simulink model "sampleModel135"  (R2021b)
settings: Solver=VariableStepAuto  StartTime=0.0  StopTime=10.0  RelTol=1e-3
undefined symbols (not defined in the file or in its folder): DiscIntNeverNeededParam, Newton, Raphson
libraries: simulink x19, slpidlib x3
settings Model: Creator=user  LastModifiedBy=user

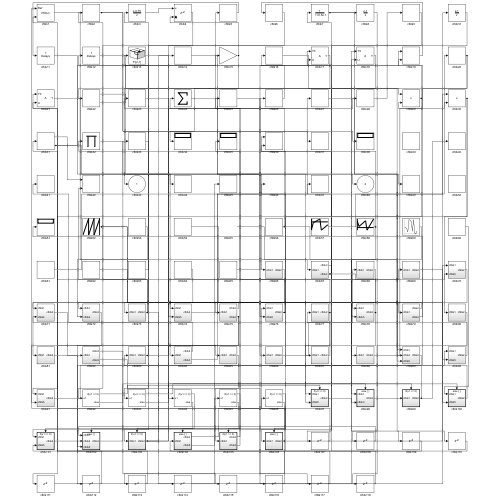
[thumbnail: Simulink's stored preview of the top-level diagram]
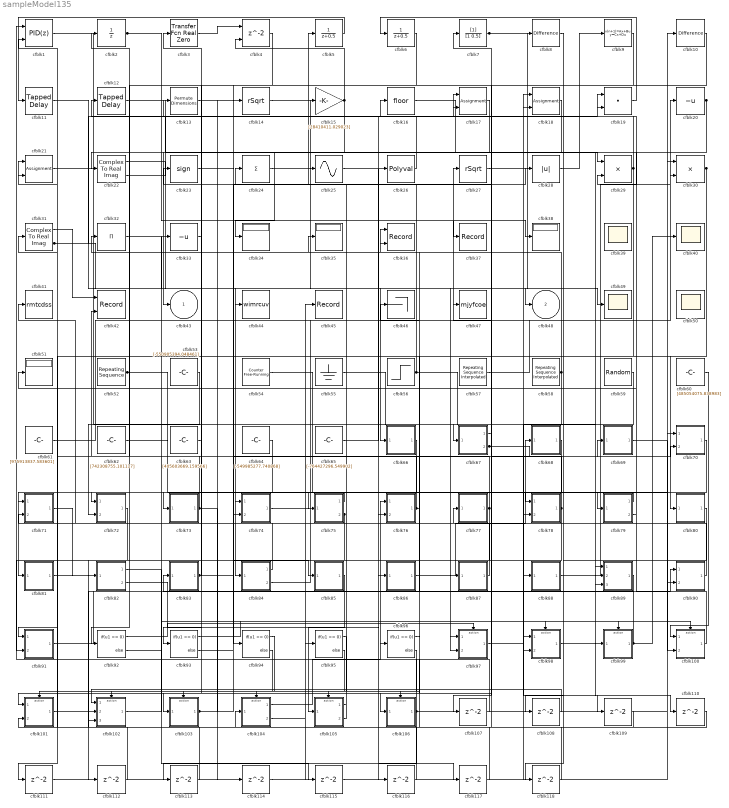
== system sampleModel135 ==
  cfblk1 : slpidlib/PID Controller (2DOF)  Controller=PID  Form=Parallel  TimeDomain=Discrete-time  UseExternalTs=off  SampleTime=1  IntegratorMethod=Forward Euler  FilterMethod=Forward Euler  ControllerParametersSource=internal  P=1  I=1  D=0  UseFilter=on  N=100  b=1  c=1  TunerSelectOption=Transfer Function Based (PID Tuner App)  InitialConditionSource=internal  InitialConditionForIntegrator=0  InitialConditionForFilter=0  DifferentiatorICPrevScaledInput=0  ExternalReset=none  TrackingMode=off  Kt=1  LimitOutput=off  SatLimitsSource=internal  UpperSaturationLimit=inf  LowerSaturationLimit=-inf  LinearizeAsGain=off  AntiWindupMode=none  Kb=1  POutMin=[]  POutMax=[]  IOutMin=[]  IOutMax=[]  DOutMin=[]  DOutMax=[]  NOutMin=[]  NOutMax=[]  bOutMin=[]  bOutMax=[]  cOutMin=[]  cOutMax=[]  SumOutMin=[]  SumOutMax=[]  SaturationOutMin=[]  SaturationOutMax=[]  PParamMin=[]  PParamMax=[]  IParamMin=[]  IParamMax=[]  DParamMin=[]  DParamMax=[]  NParamMin=[]  NParamMax=[]  bParamMin=[]  bParamMax=[]  cParamMin=[]  cParamMax=[]  KbParamMin=[]  KbParamMax=[]  KtParamMin=[]  KtParamMax=[]  KbOutMin=[]  KbOutMax=[]  KtOutMin=[]  KtOutMax=[]  IntegratorOutMin=[]  IntegratorOutMax=[]  FilterOutMin=[]  FilterOutMax=[]  SumI1OutMin=[]  SumI1OutMax=[]  SumI2OutMin=[]  SumI2OutMax=[]  SumI3OutMin=[]  SumI3OutMax=[]  SumI4OutMin=[]  SumI4OutMax=[]  SumDOutMin=[]  SumDOutMax=[]  Sum1OutMin=[]  Sum1OutMax=[]  Sum2OutMin=[]  Sum2OutMax=[]  Sum3OutMin=[]  Sum3OutMax=[]  DifferentiatorOutMin=[]  DifferentiatorOutMax=[]  FilterDiffOutCoefMin=[]  FilterDiffOutCoefMax=[]  ReciprocalOutMin=[]  ReciprocalOutMax=[]  SumDenOutMin=[]  SumDenOutMax=[]  SumNumOutMin=[]  SumNumOutMax=[]  DivideOutMin=[]  DivideOutMax=[]  UdiffTsProdOutMin=[]  UdiffTsProdOutMax=[]  NTsProdOutMin=[]  NTsProdOutMax=[]  UintegralTsProdOutMin=[]  UintegralTsProdOutMax=[]  UngainTsProdOutMin=[]  UngainTsProdOutMax=[]  IntegratorContinuousStateAttributes=''  IntegratorStateMustResolveToSignalObject=off  IntegratorRTWStateStorageClass=Auto  FilterContinuousStateAttributes=''  FilterStateMustResolveToSignalObject=off  FilterRTWStateStorageClass=Auto  ParallelPVariant=InternalParameters  IdealPVariant=Disabled  IVariant=InternalParameters  DVariant=InternalParameters  bVariant=InternalParameters  cVariant=InternalParameters  IntegratorVariant=Discrete  SatVariant=Disabled  AWVariant=Passthrough  PCopyVariant=Disabled  TRVariant=Disabled  FdbkBlocksVariant=Forward  IdealPFdbkVariant=Disabled  SatFdbkVariant=Disabled  DerivativeFilterVariant=ForwardEulerFilter  NVariant=InternalParameters  NCopyVariant=Disabled  FilterICVariant=InternalICsFilter  IntegratorICVariant=InternalICs  ExternalResetVariant=Disabled  TRSumVariant=Passthrough  SumFdbkVariant=Disabled  SumVariant=Sum_PID  TsampFilterVariant=InternalTs  TsampNgainVariant=Passthrough  TsampIntegralVariant=Passthrough  ExternalSaturationOutDataTypeStr=Inherit: Same as second input
      settings: SourceProductBaseCode=SL
  cfblk10 : simulink/Discrete/Difference  ICPrevInput=0.0  OutMin=[]  OutMax=[]  OutDataTypeStr=Inherit: Inherit via back propagation  OutDataType=fixdt(1, 16)  OutScaling=2^-10  DoSatur=off
  cfblk100 : Subsystem  TreatAsAtomicUnit=on
  cfblk101 : Subsystem  TreatAsAtomicUnit=on
  cfblk102 : Subsystem  TreatAsAtomicUnit=on
  cfblk103 : Subsystem  TreatAsAtomicUnit=on
  cfblk104 : Subsystem  TreatAsAtomicUnit=on
  cfblk105 : Subsystem  TreatAsAtomicUnit=on
  cfblk106 : Subsystem  TreatAsAtomicUnit=on
  cfblk{107..118} (12 alike) : Delay  SampleTime=1
  cfblk11 : simulink/Discrete/Tapped Delay  vinit=0.0  samptime=-1  NumDelays=1  DelayOrder=Oldest  includeCurrent=off
  cfblk12 : simulink/Discrete/Tapped Delay  vinit=0.0  samptime=-1  NumDelays=1  DelayOrder=Oldest  includeCurrent=off
  cfblk13 : PermuteDimensions
  cfblk14 : Sqrt  Operator=rSqrt  AlgorithmType=Newton-Raphson  SaturateOnIntegerOverflow=on
  cfblk15 : Gain  Gain=[28410411.029023]
  cfblk16 : Rounding
  cfblk17 : Assignment  DiagnosticForDimensions=Warning  IndexOptions=Index vector (dialog)  Indices=1  OutputSizes=1
  cfblk18 : Assignment  DiagnosticForDimensions=Warning  IndexOptions=Index vector (dialog)  Indices=1  OutputSizes=1
  cfblk19 : DotProduct  InputSameDT=on  OutDataTypeStr=Inherit: Inherit via internal rule
  cfblk2 : UnitDelay  HasFrameUpgradeWarning=on
  cfblk20 : UnaryMinus
  cfblk21 : Assignment  DiagnosticForDimensions=Warning  IndexOptions=Index vector (dialog)  Indices=1  OutputSizes=1
  cfblk22 : ComplexToRealImag
  cfblk23 : Signum
  cfblk24 : Sum  Inputs=+
  cfblk25 : Sin  TimeSource=Use external signal  SampleTime=0
  cfblk26 : Polyval  Coefs=[ +2.081618890e-019, -1.441693666e-014, +4.719686976e-010, -8.536869453e-006, +1.621573104e-001, -8.087801117e+001 ]
  cfblk27 : Sqrt  Operator=rSqrt  AlgorithmType=Newton-Raphson  SaturateOnIntegerOverflow=on
  cfblk28 : Abs
  cfblk29 : Product  Inputs=**
  cfblk3 : simulink/Discrete/Transfer Fcn Real Zero  ZeroZ=0.75  ICPrevInput=0.0  DoSatur=off
      settings: SourceProductBaseCode=SL
  cfblk30 : Product
  cfblk31 : ComplexToRealImag
  cfblk32 : Product  Inputs=*
  cfblk33 : UnaryMinus
  cfblk{34..35,38,51} (4 alike) : Display
  cfblk36 : Record  FileSettingsInternal="{\"entries\":[{\"content\":{\"excelSettings\":{\"content\":{},\"type\":\"Streamout.ExcelSettings\"}},\"type\":\"Streamout.FileSettingStorage\",\"uuid\":\"dc4603f7-060f-47ee-a389-6b2f5d8eacf3\"}],\"packageUris\":[\"http://schema.mathworks.com/mf0/streamout_blocks/R2020a\"],\"version\":\"1.0\"}"  Layout=[1 1]  SignalsInternal="{\"entries\":[{\"content\":{\"signals\":[{\"content\":{\"blockPath\":[\"sampleModel135/cfblk36\"],\"channel\":[],\"dimensions\":[1],\"domain\":\"sampleModel135/cfblk36\",\"lineColor\":\"#a2142f\",\"plots\":[1],\"port\":1,\"sid\":[\"\"],\"signalID\":4712,\"signalName\":\"cfblk76\"},\"type\":\"RecordBlkView.Signal\",\"uuid\":\"88f8ffe8-7962-43a1-8896-d692d2f87f4c\"},{\"content\":{\"blockPath\":[\"sampleModel135/cfblk36\"],\"channel\":[],\"dimensions\":[1],\"domain\":\"sampleModel135/cfblk36\",\"lineColor\":\"#139fff\",\"plots\":[1],\"port\":2,\"sid\":[\"\"],\"signalID\":4716,\"signalName\":\"cfblk67:2\"},\"type\":\"RecordBlkView.Signal\",\"uuid\":\"a67d97e2-9e96-4cb3-bdb1-be52fcd4c5cb\"}]},\"type\":\"RecordBlkView.InputSignals\",\"uuid\":\"0687f38a-ff4e-4925-8716-18ef31107799\"}],\"packageUris\":[\"http://schema.mathworks.com/mf0/streamout_blocks/R2020a\"],\"version\":\"1.0\"}"  VisualizationBindings="{\"xyplotplugin\":{\"info\":[{\"series\":[{\"bindingParametersList\":[{\"parameter\":\"X-Axis\",\"signalID\":4712,\"signalName\":\"cfblk76\"},{\"parameter\":\"Y-Axis\",\"signalID\":4716,\"signalName\":\"cfblk67:2\"}],\"seriesID\":6412}],\"subplotID\":1}]}}"  CompatibilityTag=XY
  cfblk37 : Record  FileSettingsInternal="{\"entries\":[{\"content\":{\"excelSettings\":{\"content\":{},\"type\":\"Streamout.ExcelSettings\"}},\"type\":\"Streamout.FileSettingStorage\",\"uuid\":\"5de6cc85-0c80-4659-8aff-d8a8f7568a02\"}],\"packageUris\":[\"http://schema.mathworks.com/mf0/streamout_blocks/R2020a\"],\"version\":\"1.0\"}"  SignalsInternal="{\"entries\":[{\"content\":{\"signals\":[{\"content\":{\"blockPath\":[\"sampleModel135/cfblk37\"],\"channel\":[],\"dimensions\":[1],\"domain\":\"sampleModel135/cfblk37\",\"lineColor\":\"#a2142f\",\"plots\":[1],\"port\":1,\"sid\":[\"\"],\"signalID\":4720,\"signalName\":\"cfblk2\"},\"type\":\"RecordBlkView.Signal\",\"uuid\":\"9ad653bb-3f93-4fe3-8d88-ee341a26a170\"}]},\"type\":\"RecordBlkView.InputSignals\",\"uuid\":\"e2ea3720-dc8c-4658-944f-b29d6f1fb988\"}],\"packageUris\":[\"http://schema.mathworks.com/mf0/streamout_blocks/R2020a\"],\"version\":\"1.0\"}"  VisualizationBindings="{\"sparklinesplugin\":{\"info\":[{\"bindingParametersList\":[],\"subplotID\":1}]}}"
  cfblk{39..40,49..50} (4 alike) : Scope
      cfblk39 settings: Floating=on
      cfblk50 settings: Floating=on
  cfblk4 : Delay  ShowEnablePort=on  SampleTime=1
      settings: InputPortMap=u0,e6
  cfblk41 : ToWorkspace  VariableName=rmtcdss  SaveFormat=Timeseries  SampleTime=-1
  cfblk42 : Record  FileSettingsInternal="{\"entries\":[{\"content\":{\"excelSettings\":{\"content\":{},\"type\":\"Streamout.ExcelSettings\"}},\"type\":\"Streamout.FileSettingStorage\",\"uuid\":\"3a613f90-b4b9-4c61-961a-fdb05aa120f1\"}],\"packageUris\":[\"http://schema.mathworks.com/mf0/streamout_blocks/R2020a\"],\"version\":\"1.0\"}"  Layout=[1 1]  SignalsInternal="{\"entries\":[{\"content\":{\"signals\":[{\"content\":{\"blockPath\":[\"sampleModel135/cfblk42\"],\"channel\":[],\"dimensions\":[1],\"domain\":\"sampleModel135/cfblk42\",\"lineColor\":\"#a2142f\",\"plots\":[1],\"port\":1,\"sid\":[\"\"],\"signalID\":4724,\"signalName\":\"cfblk31:1\"},\"type\":\"RecordBlkView.Signal\",\"uuid\":\"ce349fb7-b3a0-4447-98f3-427877e07b8c\"},{\"content\":{\"blockPath\":[\"sampleModel135/cfblk42\"],\"channel\":[],\"dimensions\":[1],\"domain\":\"sampleModel135/cfblk42\",\"lineColor\":\"#139fff\",\"plots\":[1],\"port\":2,\"sid\":[\"\"],\"signalID\":4728,\"signalName\":\"cfblk73\"},\"type\":\"RecordBlkView.Signal\",\"uuid\":\"6a64b2c5-78f2-443e-96fe-3bc98703bc06\"}]},\"type\":\"RecordBlkView.InputSignals\",\"uuid\":\"472f762d-471a-4371-944a-d30467dc95ae\"}],\"packageUris\":[\"http://schema.mathworks.com/mf0/streamout_blocks/R2020a\"],\"version\":\"1.0\"}"  VisualizationBindings="{\"xyplotplugin\":{\"info\":[{\"series\":[{\"bindingParametersList\":[{\"parameter\":\"X-Axis\",\"signalID\":4724,\"signalName\":\"cfblk31:1\"},{\"parameter\":\"Y-Axis\",\"signalID\":4728,\"signalName\":\"cfblk73\"}],\"seriesID\":39813}],\"subplotID\":1}]}}"  CompatibilityTag=XY
  cfblk44 : ToWorkspace  VariableName=wimrcuv  SaveFormat=Timeseries  SampleTime=-1
  cfblk45 : Record  FileSettingsInternal="{\"entries\":[{\"content\":{\"excelSettings\":{\"content\":{},\"type\":\"Streamout.ExcelSettings\"}},\"type\":\"Streamout.FileSettingStorage\",\"uuid\":\"b06d5a54-4607-4223-bf0d-fc84dbd604d8\"}],\"packageUris\":[\"http://schema.mathworks.com/mf0/streamout_blocks/R2020a\"],\"version\":\"1.0\"}"  SignalsInternal="{\"entries\":[{\"content\":{\"signals\":[{\"content\":{\"blockPath\":[\"sampleModel135/cfblk45\"],\"channel\":[],\"dimensions\":[1],\"domain\":\"sampleModel135/cfblk45\",\"lineColor\":\"#b746ff\",\"plots\":[1],\"port\":1,\"sid\":[\"\"],\"signalID\":4732,\"signalName\":\"cfblk104:2\"},\"type\":\"RecordBlkView.Signal\",\"uuid\":\"831cb24a-ecf3-4b9e-81f9-60f1a74fc749\"}]},\"type\":\"RecordBlkView.InputSignals\",\"uuid\":\"5b04a1d9-3887-4891-afc8-c46e7e218a24\"}],\"packageUris\":[\"http://schema.mathworks.com/mf0/streamout_blocks/R2020a\"],\"version\":\"1.0\"}"  VisualizationBindings="{\"sparklinesplugin\":{\"info\":[{\"bindingParametersList\":[],\"subplotID\":1}]}}"
  cfblk46 : Terminator
  cfblk47 : ToWorkspace  VariableName=mjyfcoe  SaveFormat=Timeseries  SampleTime=-1
  cfblk5 : DiscreteTransferFcn  SampleTime=1
  cfblk52 : simulink/Sources/Repeating Sequence  rep_seq_t=[0 2]  rep_seq_y=[477640940.241571, 909947082.671190]
  cfblk53 : Constant  Value=[-550905394.048461]  SampleTime=1
  cfblk54 : simulink/Sources/Counter Free-Running  NumBits=[15.000000]  tsamp=-1
  cfblk55 : Ground
  cfblk56 : Step  Time=[24.000000]  Before=[-595461991.186605]  After=[-347251148.629385]  SampleTime=0
  cfblk57 : simulink/Sources/Repeating Sequence Interpolated  OutValues=[-698628012.134013, -76558517.748631, 311619998.084971, -846087687.549569, -298956944.646346]  TimeValues=[0 0.1 0.5 0.6 1].'  LookUpMeth=Interpolation-Use End Values  tsamp=0.01  OutMin=[]  OutMax=[]  OutDataTypeStr=double  OutputDataTypeScalingMode=double  OutDataType=fixdt(0,8)  OutScaling=2^-10
  cfblk58 : simulink/Sources/Repeating Sequence Interpolated  OutValues=[752332312.195068, 107819467.006181, 768088279.352811, -288841479.675765, 972343704.108739]  TimeValues=[0 0.1 0.5 0.6 1].'  LookUpMeth=Use Input Above  tsamp=0.01  OutMin=[]  OutMax=[]  OutDataTypeStr=double  OutputDataTypeScalingMode=double  OutDataType=fixdt(0,8)  OutScaling=2^-10
  cfblk59 : RandomNumber  Mean=[72182.026536]  Variance=[16955.399432]  Seed=[307408944.000000]  SampleTime=0.1
  cfblk6 : DiscreteTransferFcn  SampleTime=1
  cfblk60 : Constant  Value=[485054075.838983]  SampleTime=1
  cfblk61 : Constant  Value=[975913837.583601]  SampleTime=1
  cfblk62 : Constant  Value=[742308755.101117]  SampleTime=1
  cfblk63 : Constant  Value=[405603669.159566]  SampleTime=1
  cfblk64 : Constant  Value=[-549985277.740868]  SampleTime=1
  cfblk65 : Constant  Value=[-764427296.549902]  SampleTime=1
  cfblk66 : Subsystem
  cfblk67 : Subsystem
  cfblk68 : Subsystem
  cfblk69 : Subsystem
  cfblk7 : DiscreteFilter  SampleTime=1
  cfblk70 : Subsystem
  cfblk71 : Subsystem
  cfblk72 : Subsystem
  cfblk73 : Subsystem
  cfblk74 : Subsystem
  cfblk75 : Subsystem
  cfblk76 : Subsystem
  cfblk77 : Subsystem
  cfblk78 : Subsystem
  cfblk79 : Subsystem
  cfblk8 : simulink/Discrete/Difference  ICPrevInput=0.0  OutMin=[]  OutMax=[]  OutDataTypeStr=Inherit: Inherit via back propagation  OutDataType=fixdt(1, 16)  OutScaling=2^-10  DoSatur=off
  cfblk80 : Subsystem
  cfblk81 : Subsystem
  cfblk82 : Subsystem
  cfblk83 : Subsystem
  cfblk84 : Subsystem
  cfblk85 : Subsystem
  cfblk86 : Subsystem
  cfblk87 : Subsystem
  cfblk88 : Subsystem
  cfblk89 : Subsystem
  cfblk9 : DiscreteStateSpace
  cfblk90 : Subsystem
  cfblk91 : Subsystem
  cfblk{92..96} (5 alike) : If  IfExpression=u1 >= 0  SampleTime=1
  cfblk97 : Subsystem  TreatAsAtomicUnit=on
  cfblk98 : Subsystem  TreatAsAtomicUnit=on
  cfblk99 : Subsystem  TreatAsAtomicUnit=on
  cfblk43 : Outport
  cfblk48 : Outport  Port=2
  wires:
  cfblk71/1(cfblk2) -> cfblk82/1(cfblk1)
  cfblk17/1 -> cfblk43/1
  cfblk28/1 -> cfblk9/1
  cfblk18/1 -> cfblk24/1
  cfblk84/1(cfblk2) -> cfblk41/1
  cfblk15/1 -> cfblk34/1, cfblk4/2
  cfblk89/1(cfblk2) -> cfblk83/1(cfblk1)
  cfblk85/1(cfblk2) -> cfblk105/1(cfblk1)
  cfblk1/1 -> cfblk67/1(cfblk1)
  cfblk5/1 -> cfblk11/1
  cfblk19/1 -> cfblk6/1
  cfblk90/1(cfblk2) -> cfblk77/1(cfblk1)
  cfblk68/1(cfblk2) -> cfblk81/1(cfblk1)
  cfblk61/1 -> cfblk27/1
  cfblk12/1 -> cfblk29/1
  cfblk56/1 -> cfblk5/1, cfblk89/3(cfblk5)
  cfblk101/1(cfblk2) -> cfblk90/1(cfblk1)
  cfblk13/1 -> cfblk94/1
  cfblk22/1 -> cfblk84/1(cfblk1)
  cfblk83/1(cfblk2) -> cfblk3/1, cfblk85/1(cfblk1)
  cfblk64/1 -> cfblk72/1(cfblk1)
  cfblk62/1 -> cfblk97/1(cfblk1)
  cfblk104/1(cfblk2) -> cfblk76/1(cfblk1)
  cfblk30/1 -> cfblk80/1(cfblk1), cfblk111/1
  cfblk20/1 -> cfblk29/2, cfblk22/1
  cfblk86/1(cfblk2) -> cfblk68/1(cfblk1)
  cfblk53/1 -> cfblk72/2(cfblk4)
  cfblk102/1(cfblk2) -> cfblk33/1
  cfblk29/1 -> cfblk16/1, cfblk106/1(cfblk1)
  cfblk88/1(cfblk2) -> cfblk20/1
  cfblk104/2(cfblk5) -> cfblk45/1
  cfblk16/1 -> cfblk99/1(cfblk1)
  cfblk31/1 -> cfblk42/1
  cfblk21/1 -> cfblk87/1(cfblk1)
  cfblk23/1 -> cfblk79/1(cfblk1)
  cfblk66/1(cfblk2) -> cfblk71/1(cfblk1)
  cfblk73/1(cfblk2) -> cfblk12/1, cfblk42/2, cfblk114/1
  cfblk60/1 -> cfblk100/1(cfblk1)
  cfblk11/1 -> cfblk44/1
  cfblk52/1 -> cfblk76/2(cfblk5), cfblk98/1(cfblk1)
  cfblk24/1 -> cfblk66/1(cfblk1)
  cfblk14/1 -> cfblk48/1
  cfblk106/1(cfblk2) -> cfblk30/1, cfblk21/1, cfblk113/1
  cfblk76/1(cfblk2) -> cfblk36/1, cfblk35/1
  cfblk63/1 -> cfblk13/1
  cfblk27/1 -> cfblk89/1(cfblk1)
  cfblk100/1(cfblk2) -> cfblk19/1
  cfblk33/1 -> cfblk93/1
  cfblk78/1(cfblk2) -> cfblk97/2(cfblk5), cfblk47/1
  cfblk22/2 -> cfblk15/1
  cfblk105/1(cfblk2) -> cfblk25/1
  cfblk67/1(cfblk2) -> cfblk101/1(cfblk1)
  cfblk74/1(cfblk2) -> cfblk10/1
  cfblk99/1(cfblk2) -> cfblk46/1, cfblk40/1
  cfblk7/1 -> cfblk89/2(cfblk4), cfblk8/1
  cfblk79/1(cfblk2) -> cfblk78/1(cfblk1)
  cfblk67/2(cfblk4) -> cfblk36/2, cfblk69/1(cfblk1), cfblk17/2
  cfblk57/1 -> cfblk30/2
  cfblk72/1(cfblk2) -> cfblk102/3(cfblk5)
  cfblk69/1(cfblk2) -> cfblk90/2(cfblk5)
  cfblk84/2(cfblk3) -> cfblk26/1
  cfblk91/1(cfblk2) -> cfblk18/1
  cfblk105/2(cfblk4) -> cfblk23/1
  cfblk10/1 -> cfblk73/1(cfblk1)
  cfblk79/2(cfblk4) -> cfblk51/1
  cfblk75/1(cfblk2) -> cfblk74/1(cfblk1)
  cfblk26/1 -> cfblk2/1
  cfblk3/1 -> cfblk4/1
  cfblk2/1 -> cfblk37/1, cfblk38/1
  cfblk87/1(cfblk2) -> cfblk31/1
  cfblk4/1 -> cfblk74/2(cfblk5)
  cfblk31/2 -> cfblk86/1(cfblk1), cfblk19/2
  cfblk70/1(cfblk2) -> cfblk75/1(cfblk1)
  cfblk75/2(cfblk4) -> cfblk91/1(cfblk1), cfblk91/2(cfblk5)
  cfblk77/1(cfblk2) -> cfblk103/1(cfblk1), cfblk21/2
  cfblk55/1 -> cfblk88/1(cfblk1)
  cfblk58/1 -> cfblk32/1, cfblk98/2(cfblk3)
  cfblk54/1 -> cfblk100/2(cfblk5)
  cfblk6/1 -> cfblk92/1
  cfblk59/1 -> cfblk78/2(cfblk5)
  cfblk103/1(cfblk2) -> cfblk28/1, cfblk14/1, cfblk70/2(cfblk5)
  cfblk32/1 -> cfblk49/1
  cfblk65/1 -> cfblk17/1
  cfblk92/1 -> cfblk97/Action
  cfblk92/2 -> cfblk98/Action
  cfblk93/1 -> cfblk99/Action
  cfblk93/2 -> cfblk100/Action
  cfblk94/1 -> cfblk101/Action
  cfblk94/2 -> cfblk102/Action
  cfblk95/1 -> cfblk103/Action
  cfblk95/2 -> cfblk104/Action
  cfblk96/1 -> cfblk105/Action
  cfblk96/2 -> cfblk106/Action
  cfblk9/1 -> cfblk107/1
  cfblk107/1 -> cfblk1/1
  cfblk80/1(cfblk2) -> cfblk108/1
  cfblk108/1 -> cfblk102/1(cfblk1)
  cfblk97/1(cfblk2) -> cfblk109/1
  cfblk109/1 -> cfblk101/2(cfblk5)
  cfblk98/1(cfblk2) -> cfblk110/1
  cfblk110/1 -> cfblk104/1(cfblk1)
  cfblk111/1 -> cfblk95/1
  cfblk81/1(cfblk2) -> cfblk112/1
  cfblk112/1 -> cfblk102/2(cfblk4)
  cfblk113/1 -> cfblk1/2
  cfblk114/1 -> cfblk70/1(cfblk1)
  cfblk82/1(cfblk2) -> cfblk115/1
  cfblk115/1 -> cfblk18/2
  cfblk82/2(cfblk5) -> cfblk116/1
  cfblk116/1 -> cfblk71/2(cfblk4)
  cfblk25/1 -> cfblk117/1
  cfblk117/1 -> cfblk96/1
  cfblk8/1 -> cfblk118/1
  cfblk118/1 -> cfblk7/1

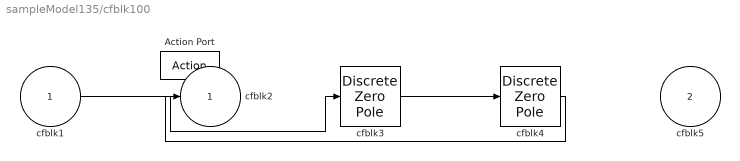
== system sampleModel135/cfblk100 ==
  cfblk1 : Inport
  cfblk5 : Inport  Port=2
  Action Port : ActionPort  ActionPortLabel=else
  cfblk3 : DiscreteZeroPole  Poles=[0 0.5]  Gain=1  SampleTime=-1
  cfblk4 : DiscreteZeroPole  Poles=[0 0.5]  Gain=1  SampleTime=-1
  cfblk2 : Outport
  wires:
  cfblk3/1 -> cfblk4/1
  cfblk1/1 -> cfblk3/1
  cfblk4/1 -> cfblk2/1

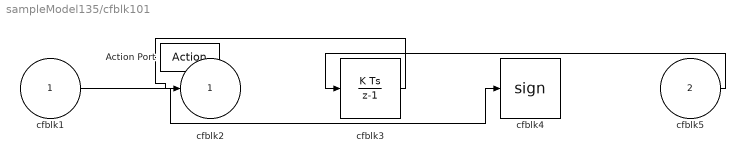
== system sampleModel135/cfblk101 ==
  cfblk1 : Inport
  cfblk5 : Inport  Port=2
  Action Port : ActionPort  ActionPortLabel=if(u1 >= 0)
  cfblk3 : DiscreteIntegrator  SampleTime=-1  ICPrevOutput=DiscIntNeverNeededParam  ICPrevScaledInput=DiscIntNeverNeededParam
  cfblk4 : Signum
  cfblk2 : Outport
  wires:
  cfblk1/1 -> cfblk4/1
  cfblk3/1 -> cfblk2/1
  cfblk5/1 -> cfblk3/1

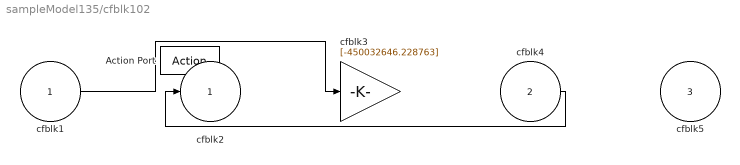
== system sampleModel135/cfblk102 ==
  cfblk1 : Inport
  cfblk4 : Inport  Port=2
  cfblk5 : Inport  Port=3
  Action Port : ActionPort  ActionPortLabel=else
  cfblk3 : Gain  Gain=[-450032646.228763]
  cfblk2 : Outport
  wires:
  cfblk4/1 -> cfblk2/1
  cfblk1/1 -> cfblk3/1

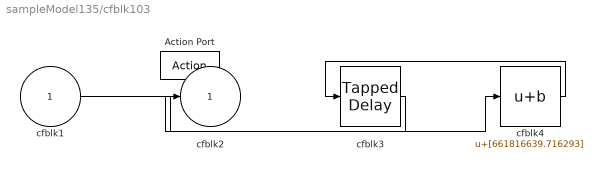
== system sampleModel135/cfblk103 ==
  cfblk1 : Inport
  Action Port : ActionPort  ActionPortLabel=if(u1 >= 0)
  cfblk3 : simulink/Discrete/Tapped Delay  vinit=0.0  samptime=-1  NumDelays=1  DelayOrder=Oldest  includeCurrent=off
  cfblk4 : Bias  Bias=[661816639.716293]
  cfblk2 : Outport
  wires:
  cfblk1/1 -> cfblk4/1
  cfblk4/1 -> cfblk3/1
  cfblk3/1 -> cfblk2/1

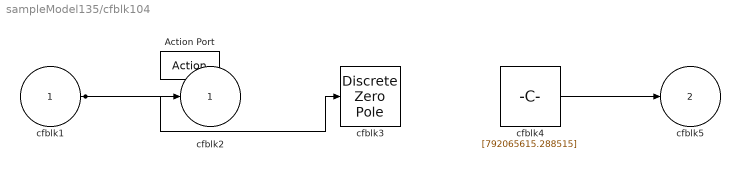
== system sampleModel135/cfblk104 ==
  cfblk1 : Inport
  Action Port : ActionPort  ActionPortLabel=else
  cfblk3 : DiscreteZeroPole  Poles=[0 0.5]  Gain=1  SampleTime=-1
  cfblk4 : Constant  Value=[792065615.288515]  SampleTime=1
  cfblk2 : Outport
  cfblk5 : Outport  Port=2
  wires:
  cfblk4/1 -> cfblk5/1
  cfblk1/1 -> cfblk2/1, cfblk3/1

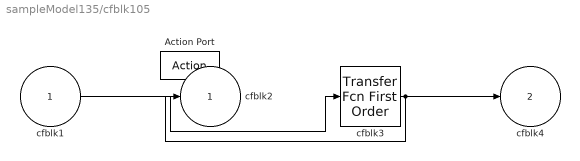
== system sampleModel135/cfblk105 ==
  cfblk1 : Inport
  Action Port : ActionPort  ActionPortLabel=if(u1 >= 0)
  cfblk3 : simulink/Discrete/Transfer Fcn First Order  PoleZ=0.95  ICPrevOutput=0.0  DoSatur=off
  cfblk2 : Outport
  cfblk4 : Outport  Port=2
  wires:
  cfblk1/1 -> cfblk3/1
  cfblk3/1 -> cfblk2/1, cfblk4/1

== system sampleModel135/cfblk106 ==
  cfblk1 : Inport
  Action Port : ActionPort  ActionPortLabel=else
  cfblk3 : ComplexToMagnitudeAngle
  cfblk2 : Outport
  wires:
  cfblk1/1 -> cfblk2/1, cfblk3/1

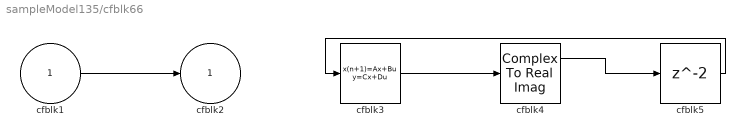
== system sampleModel135/cfblk66 ==
  cfblk1 : Inport
  cfblk3 : DiscreteStateSpace
  cfblk4 : ComplexToRealImag
  cfblk5 : Delay  SampleTime=1
  cfblk2 : Outport
  wires:
  cfblk3/1 -> cfblk4/1
  cfblk1/1 -> cfblk2/1
  cfblk4/1 -> cfblk5/1
  cfblk5/1 -> cfblk3/1

== system sampleModel135/cfblk67 ==
  cfblk1 : Inport
  cfblk3 : DiscreteStateSpace
  cfblk2 : Outport
  cfblk4 : Outport  Port=2
  wires:
  cfblk1/1 -> cfblk4/1, cfblk3/1
  cfblk3/1 -> cfblk2/1

== system sampleModel135/cfblk68 ==
  cfblk1 : Inport
  cfblk3 : DiscreteFilter  SampleTime=1
  cfblk4 : DiscreteFilter  SampleTime=1
  cfblk2 : Outport
  wires:
  cfblk4/1 -> cfblk3/1
  cfblk1/1 -> cfblk4/1
  cfblk3/1 -> cfblk2/1

== system sampleModel135/cfblk69 ==
  cfblk1 : Inport
  cfblk3 : Delay  DelayLengthSource=Input port  SampleTime=1
      settings: InputPortMap=u0,p1
  cfblk2 : Outport
  wires:
  cfblk1/1 -> cfblk3/1, cfblk3/2
  cfblk3/1 -> cfblk2/1

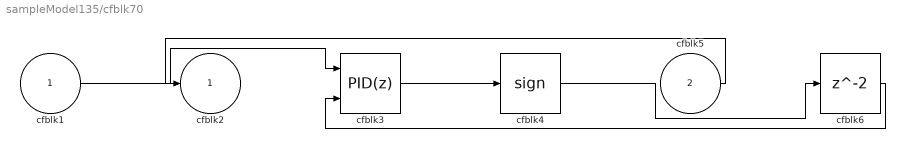
== system sampleModel135/cfblk70 ==
  cfblk1 : Inport
  cfblk5 : Inport  Port=2
  cfblk3 : slpidlib/PID Controller (2DOF)  Controller=PID  Form=Parallel  TimeDomain=Discrete-time  UseExternalTs=off  SampleTime=1  IntegratorMethod=Forward Euler  FilterMethod=Forward Euler  ControllerParametersSource=internal  P=1  I=1  D=0  UseFilter=on  N=100  b=1  c=1  TunerSelectOption=Transfer Function Based (PID Tuner App)  InitialConditionSource=internal  InitialConditionForIntegrator=0  InitialConditionForFilter=0  DifferentiatorICPrevScaledInput=0  ExternalReset=none  TrackingMode=off  Kt=1  LimitOutput=off  SatLimitsSource=internal  UpperSaturationLimit=inf  LowerSaturationLimit=-inf  LinearizeAsGain=off  AntiWindupMode=none  Kb=1  POutMin=[]  POutMax=[]  IOutMin=[]  IOutMax=[]  DOutMin=[]  DOutMax=[]  NOutMin=[]  NOutMax=[]  bOutMin=[]  bOutMax=[]  cOutMin=[]  cOutMax=[]  SumOutMin=[]  SumOutMax=[]  SaturationOutMin=[]  SaturationOutMax=[]  PParamMin=[]  PParamMax=[]  IParamMin=[]  IParamMax=[]  DParamMin=[]  DParamMax=[]  NParamMin=[]  NParamMax=[]  bParamMin=[]  bParamMax=[]  cParamMin=[]  cParamMax=[]  KbParamMin=[]  KbParamMax=[]  KtParamMin=[]  KtParamMax=[]  KbOutMin=[]  KbOutMax=[]  KtOutMin=[]  KtOutMax=[]  IntegratorOutMin=[]  IntegratorOutMax=[]  FilterOutMin=[]  FilterOutMax=[]  SumI1OutMin=[]  SumI1OutMax=[]  SumI2OutMin=[]  SumI2OutMax=[]  SumI3OutMin=[]  SumI3OutMax=[]  SumI4OutMin=[]  SumI4OutMax=[]  SumDOutMin=[]  SumDOutMax=[]  Sum1OutMin=[]  Sum1OutMax=[]  Sum2OutMin=[]  Sum2OutMax=[]  Sum3OutMin=[]  Sum3OutMax=[]  DifferentiatorOutMin=[]  DifferentiatorOutMax=[]  FilterDiffOutCoefMin=[]  FilterDiffOutCoefMax=[]  ReciprocalOutMin=[]  ReciprocalOutMax=[]  SumDenOutMin=[]  SumDenOutMax=[]  SumNumOutMin=[]  SumNumOutMax=[]  DivideOutMin=[]  DivideOutMax=[]  UdiffTsProdOutMin=[]  UdiffTsProdOutMax=[]  NTsProdOutMin=[]  NTsProdOutMax=[]  UintegralTsProdOutMin=[]  UintegralTsProdOutMax=[]  UngainTsProdOutMin=[]  UngainTsProdOutMax=[]  IntegratorContinuousStateAttributes=''  IntegratorStateMustResolveToSignalObject=off  IntegratorRTWStateStorageClass=Auto  FilterContinuousStateAttributes=''  FilterStateMustResolveToSignalObject=off  FilterRTWStateStorageClass=Auto  ParallelPVariant=InternalParameters  IdealPVariant=Disabled  IVariant=InternalParameters  DVariant=InternalParameters  bVariant=InternalParameters  cVariant=InternalParameters  IntegratorVariant=Discrete  SatVariant=Disabled  AWVariant=Passthrough  PCopyVariant=Disabled  TRVariant=Disabled  FdbkBlocksVariant=Forward  IdealPFdbkVariant=Disabled  SatFdbkVariant=Disabled  DerivativeFilterVariant=ForwardEulerFilter  NVariant=InternalParameters  NCopyVariant=Disabled  FilterICVariant=InternalICsFilter  IntegratorICVariant=InternalICs  ExternalResetVariant=Disabled  TRSumVariant=Passthrough  SumFdbkVariant=Disabled  SumVariant=Sum_PID  TsampFilterVariant=InternalTs  TsampNgainVariant=Passthrough  TsampIntegralVariant=Passthrough  ExternalSaturationOutDataTypeStr=Inherit: Same as second input
      settings: SourceProductBaseCode=SL
  cfblk4 : Signum
  cfblk6 : Delay  SampleTime=1
  cfblk2 : Outport
  wires:
  cfblk1/1 -> cfblk3/1
  cfblk3/1 -> cfblk4/1
  cfblk5/1 -> cfblk2/1
  cfblk4/1 -> cfblk6/1
  cfblk6/1 -> cfblk3/2

== system sampleModel135/cfblk71 ==
  cfblk1 : Inport
  cfblk4 : Inport  Port=2
  cfblk3 : Product
  cfblk2 : Outport
  wires:
  cfblk1/1 -> cfblk3/1, cfblk3/2
  cfblk4/1 -> cfblk2/1

== system sampleModel135/cfblk72 ==
  cfblk1 : Inport
  cfblk4 : Inport  Port=2
  cfblk3 : simulink/Discrete/Transfer Fcn Real Zero  ZeroZ=0.75  ICPrevInput=0.0  DoSatur=off
      settings: SourceProductBaseCode=SL
  cfblk2 : Outport
  wires:
  cfblk4/1 -> cfblk3/1
  cfblk1/1 -> cfblk2/1

== system sampleModel135/cfblk73 ==
  cfblk1 : Inport
  cfblk3 : Gain  Gain=[-521772301.207292]
  cfblk4 : Constant  Value=[-65790719.419263]  SampleTime=1
  cfblk2 : Outport
  wires:
  cfblk1/1 -> cfblk3/1
  cfblk4/1 -> cfblk2/1

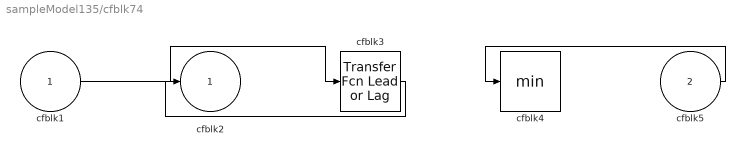
== system sampleModel135/cfblk74 ==
  cfblk1 : Inport
  cfblk5 : Inport  Port=2
  cfblk3 : simulink/Discrete/Transfer Fcn Lead or Lag  PoleZ=0.95  ZeroZ=0.75  ICPrevOutput=0.0  ICPrevInput=0.0  DoSatur=off
      settings: SourceProductBaseCode=SL
  cfblk4 : MinMax
  cfblk2 : Outport
  wires:
  cfblk1/1 -> cfblk3/1
  cfblk3/1 -> cfblk2/1
  cfblk5/1 -> cfblk4/1

== system sampleModel135/cfblk75 ==
  cfblk1 : Inport
  cfblk3 : Sin  TimeSource=Use external signal  SampleTime=0
  cfblk2 : Outport
  cfblk4 : Outport  Port=2
  wires:
  cfblk3/1 -> cfblk4/1
  cfblk1/1 -> cfblk2/1, cfblk3/1

== system sampleModel135/cfblk76 ==
  cfblk1 : Inport
  cfblk5 : Inport  Port=2
  cfblk3 : Polyval  Coefs=[ +2.081618890e-019, -1.441693666e-014, +4.719686976e-010, -8.536869453e-006, +1.621573104e-001, -8.087801117e+001 ]
  cfblk4 : Constant  Value=[-338113701.827944]  SampleTime=1
  cfblk2 : Outport
  wires:
  cfblk4/1 -> cfblk3/1
  cfblk3/1 -> cfblk2/1

== system sampleModel135/cfblk77 ==
  cfblk1 : Inport
  cfblk3 : simulink/Discrete/Difference  ICPrevInput=0.0  OutMin=[]  OutMax=[]  OutDataTypeStr=Inherit: Inherit via back propagation  OutDataType=fixdt(1, 16)  OutScaling=2^-10  DoSatur=off
  cfblk2 : Outport
  wires:
  cfblk1/1 -> cfblk3/1
  cfblk3/1 -> cfblk2/1

== system sampleModel135/cfblk78 ==
  cfblk1 : Inport
  cfblk5 : Inport  Port=2
  cfblk3 : ComplexToRealImag
  cfblk4 : ComplexToMagnitudeAngle
  cfblk2 : Outport
  wires:
  cfblk3/1 -> cfblk2/1
  cfblk1/1 -> cfblk4/1
  cfblk4/1 -> cfblk3/1

== system sampleModel135/cfblk79 ==
  cfblk1 : Inport
  cfblk3 : DiscreteFir  SampleTime=1
  cfblk2 : Outport
  cfblk4 : Outport  Port=2
  wires:
  cfblk1/1 -> cfblk4/1, cfblk3/1
  cfblk3/1 -> cfblk2/1

== system sampleModel135/cfblk80 ==
  cfblk1 : Inport
  cfblk3 : Gain  Gain=[-235992841.501471]
  cfblk2 : Outport
  wires:
  cfblk1/1 -> cfblk3/1
  cfblk3/1 -> cfblk2/1

== system sampleModel135/cfblk81 ==
  cfblk1 : Inport
  cfblk3 : Sum  Inputs=+-
  cfblk2 : Outport
  wires:
  cfblk1/1 -> cfblk2/1, cfblk3/1, cfblk3/2

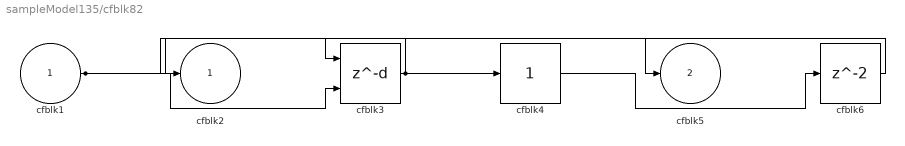
== system sampleModel135/cfblk82 ==
  cfblk1 : Inport
  cfblk3 : Delay  DelayLengthSource=Input port  SampleTime=1
      settings: InputPortMap=u0,p1
  cfblk4 : simulink/Math Operations/Slider Gain  gain=1  low=0  high=2
  cfblk6 : Delay  SampleTime=1
  cfblk2 : Outport
  cfblk5 : Outport  Port=2
  wires:
  cfblk3/1 -> cfblk4/1, cfblk2/1
  cfblk1/1 -> cfblk3/2, cfblk5/1
  cfblk4/1 -> cfblk6/1
  cfblk6/1 -> cfblk3/1

== system sampleModel135/cfblk83 ==
  cfblk1 : Inport
  cfblk3 : Sum  Inputs=|++
  cfblk4 : Constant  Value=[749133548.970775]  SampleTime=1
  cfblk2 : Outport
  wires:
  cfblk4/1 -> cfblk3/1
  cfblk1/1 -> cfblk3/2
  cfblk3/1 -> cfblk2/1

== system sampleModel135/cfblk84 ==
  cfblk1 : Inport
  cfblk2 : Outport
  cfblk3 : Outport  Port=2
  wires:
  cfblk1/1 -> cfblk3/1, cfblk2/1

== system sampleModel135/cfblk85 ==
  cfblk1 : Inport
  cfblk3 : DiscreteTransferFcn  SampleTime=1
  cfblk4 : PermuteDimensions
  cfblk2 : Outport
  wires:
  cfblk3/1 -> cfblk2/1, cfblk4/1
  cfblk1/1 -> cfblk3/1

== system sampleModel135/cfblk86 ==
  cfblk1 : Inport
  cfblk3 : Delay  DelayLengthSource=Input port  SampleTime=1
      settings: InputPortMap=u0,p1
  cfblk4 : Trigonometry
  cfblk5 : simulink/Math Operations/Slider Gain  gain=1  low=0  high=2
  cfblk2 : Outport
  wires:
  cfblk4/1 -> cfblk2/1
  cfblk1/1 -> cfblk3/1, cfblk5/1
  cfblk5/1 -> cfblk3/2
  cfblk3/1 -> cfblk4/1

== system sampleModel135/cfblk87 ==
  cfblk1 : Inport
  cfblk3 : simulink/Discrete/Tapped Delay  vinit=0.0  samptime=-1  NumDelays=1  DelayOrder=Oldest  includeCurrent=off
  cfblk2 : Outport
  wires:
  cfblk3/1 -> cfblk2/1
  cfblk1/1 -> cfblk3/1

== system sampleModel135/cfblk88 ==
  cfblk1 : Inport
  cfblk3 : simulink/Discrete/Transfer Fcn Real Zero  ZeroZ=0.75  ICPrevInput=0.0  DoSatur=off
      settings: SourceProductBaseCode=SL
  cfblk2 : Outport
  wires:
  cfblk1/1 -> cfblk3/1
  cfblk3/1 -> cfblk2/1

== system sampleModel135/cfblk89 ==
  cfblk1 : Inport
  cfblk4 : Inport  Port=2
  cfblk5 : Inport  Port=3
  cfblk3 : Constant  Value=[548910403.569160]  SampleTime=1
  cfblk2 : Outport
  wires:
  cfblk1/1 -> cfblk2/1

== system sampleModel135/cfblk90 ==
  cfblk1 : Inport
  cfblk5 : Inport  Port=2
  cfblk3 : simulink/Discrete/Difference  ICPrevInput=0.0  OutMin=[]  OutMax=[]  OutDataTypeStr=Inherit: Inherit via back propagation  OutDataType=fixdt(1, 16)  OutScaling=2^-10  DoSatur=off
  cfblk4 : slpidlib/PID Controller  Controller=PID  Form=Parallel  TimeDomain=Discrete-time  UseExternalTs=off  SampleTime=1  IntegratorMethod=Forward Euler  FilterMethod=Forward Euler  ControllerParametersSource=internal  P=1  I=1  D=0  UseFilter=on  N=100  TunerSelectOption=Transfer Function Based (PID Tuner App)  InitialConditionSource=internal  InitialConditionForIntegrator=0  InitialConditionForFilter=0  DifferentiatorICPrevScaledInput=0  ExternalReset=none  TrackingMode=off  Kt=1  LimitOutput=off  SatLimitsSource=internal  UpperSaturationLimit=inf  LowerSaturationLimit=-inf  LinearizeAsGain=off  AntiWindupMode=none  Kb=1  POutMin=[]  POutMax=[]  IOutMin=[]  IOutMax=[]  DOutMin=[]  DOutMax=[]  NOutMin=[]  NOutMax=[]  SumOutMin=[]  SumOutMax=[]  SaturationOutMin=[]  SaturationOutMax=[]  PParamMin=[]  PParamMax=[]  IParamMin=[]  IParamMax=[]  DParamMin=[]  DParamMax=[]  NParamMin=[]  NParamMax=[]  KbParamMin=[]  KbParamMax=[]  KtParamMin=[]  KtParamMax=[]  KbOutMin=[]  KbOutMax=[]  KtOutMin=[]  KtOutMax=[]  IntegratorOutMin=[]  IntegratorOutMax=[]  FilterOutMin=[]  FilterOutMax=[]  SumI1OutMin=[]  SumI1OutMax=[]  SumI2OutMin=[]  SumI2OutMax=[]  SumI3OutMin=[]  SumI3OutMax=[]  SumI4OutMin=[]  SumI4OutMax=[]  SumDOutMin=[]  SumDOutMax=[]  DifferentiatorOutMin=[]  DifferentiatorOutMax=[]  FilterDiffOutCoefMin=[]  FilterDiffOutCoefMax=[]  ReciprocalOutMin=[]  ReciprocalOutMax=[]  SumDenOutMin=[]  SumDenOutMax=[]  SumNumOutMin=[]  SumNumOutMax=[]  DivideOutMin=[]  DivideOutMax=[]  UdiffTsProdOutMin=[]  UdiffTsProdOutMax=[]  NTsProdOutMin=[]  NTsProdOutMax=[]  UintegralTsProdOutMin=[]  UintegralTsProdOutMax=[]  UngainTsProdOutMin=[]  UngainTsProdOutMax=[]  IntegratorContinuousStateAttributes=''  IntegratorStateMustResolveToSignalObject=off  IntegratorRTWStateStorageClass=Auto  FilterContinuousStateAttributes=''  FilterStateMustResolveToSignalObject=off  FilterRTWStateStorageClass=Auto  ParallelPVariant=InternalParameters  IdealPVariant=Disabled  IVariant=InternalParameters  DVariant=InternalParameters  IntegratorVariant=Discrete  SatVariant=Disabled  AWVariant=Passthrough  PCopyVariant=Disabled  TRVariant=Disabled  FdbkBlocksVariant=Forward  IdealPFdbkVariant=Disabled  SatFdbkVariant=Disabled  DerivativeFilterVariant=ForwardEulerFilter  NVariant=InternalParameters  NCopyVariant=Disabled  FilterICVariant=InternalICsFilter  IntegratorICVariant=InternalICs  ExternalResetVariant=Disabled  TRSumVariant=Passthrough  SumFdbkVariant=Disabled  SumVariant=Sum_PID  TsampFilterVariant=InternalTs  TsampNgainVariant=Passthrough  TsampIntegralVariant=Passthrough  ExternalSaturationOutDataTypeStr=Inherit: Same as second input
  cfblk2 : Outport
  wires:
  cfblk3/1 -> cfblk2/1
  cfblk1/1 -> cfblk4/1
  cfblk4/1 -> cfblk3/1

== system sampleModel135/cfblk91 ==
  cfblk1 : Inport
  cfblk5 : Inport  Port=2
  cfblk3 : Constant  Value=[710884166.295395]  SampleTime=1
  cfblk4 : Constant  Value=[-397403311.227990]  SampleTime=1
  cfblk2 : Outport
  wires:
  cfblk3/1 -> cfblk2/1

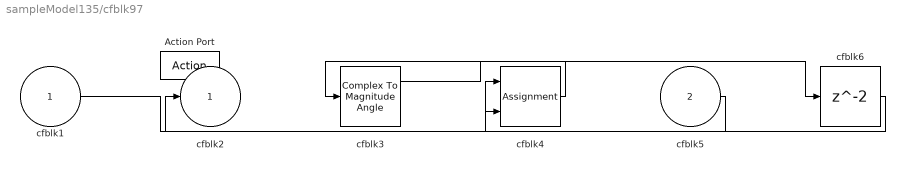
== system sampleModel135/cfblk97 ==
  cfblk1 : Inport
  cfblk5 : Inport  Port=2
  Action Port : ActionPort  ActionPortLabel=if(u1 >= 0)
  cfblk3 : ComplexToMagnitudeAngle
  cfblk4 : Assignment  DiagnosticForDimensions=Warning  IndexOptions=Index vector (dialog)  Indices=1  OutputSizes=1
  cfblk6 : Delay
  cfblk2 : Outport
  wires:
  cfblk5/1 -> cfblk2/1
  cfblk4/1 -> cfblk3/1
  cfblk1/1 -> cfblk4/1
  cfblk3/1 -> cfblk6/1
  cfblk6/1 -> cfblk4/2

== system sampleModel135/cfblk98 ==
  cfblk1 : Inport
  cfblk3 : Inport  Port=2
  Action Port : ActionPort  ActionPortLabel=else
  cfblk2 : Outport
  wires:
  cfblk1/1 -> cfblk2/1

== system sampleModel135/cfblk99 ==
  cfblk1 : Inport
  Action Port : ActionPort  ActionPortLabel=if(u1 >= 0)
  cfblk3 : Constant  Value=[-548088968.937660]  SampleTime=1
  cfblk2 : Outport
  wires:
  cfblk3/1 -> cfblk2/1
